simulink subsystem "PvtSubSys_VSM_LCKIE"  (R2020b)
settings: Solver=VariableStepAuto  StartTime=0.0  StopTime=10.0  RelTol=1e-3
values from neighbouring files (symbols this model uses):
  P_VSM_LCKIE_ClassInput = 0.0    [LCKIE.sldd]
  P_VSM_LCKIE_Laneoffset : value not decoded    [LCKIE.sldd]
  P_VSM_LCKIE_Laneoffset_BP : value not decoded    [LCKIE.sldd]
  P_VSM_LCKIE_LatC_DisOffofLanWidth : value not decoded    [LCKIE.sldd]
  P_VSM_LCKIE_LatC_DisOffofSpd : value not decoded    [LCKIE.sldd]
  P_VSM_LCKIE_LatC_DisSW = 0.0    [LCKIE.sldd]
  P_VSM_LCKIE_LatC_LanWidth : value not decoded    [LCKIE.sldd]
  P_VSM_LCKIE_LATC_LimitDis : value not decoded    [LCKIE.sldd]
  P_VSM_LCKIE_LATC_LimitDis_BP : value not decoded    [LCKIE.sldd]
  P_VSM_LCKIE_LatC_LimitDisEgoToObjSelt = 1.5    [LCKIE.sldd]
  P_VSM_LCKIE_LatC_LimitEgoToOppLane = 0.3    [LCKIE.sldd]
  P_VSM_LCKIE_LatC_maxLimitDisREToLane = 2.5    [LCKIE.sldd]
  P_VSM_LCKIE_LatC_minLimitDisREToLane = 1.2    [LCKIE.sldd]
  P_VSM_LCKIE_LatC_MoveEnableDis = 0.0    [LCKIE.sldd]
  P_VSM_LCKIE_LatC_RESafDis = 0.8    [LCKIE.sldd]
  P_VSM_LCKIE_LatC_SafeDisofLanWidth : value not decoded    [LCKIE.sldd]
  P_VSM_LCKIE_LatC_Spd : value not decoded    [LCKIE.sldd]
  P_VSM_LCKIE_LongC_d1 : value not decoded    [LCKIE.sldd]
  P_VSM_LCKIE_LongC_d2 : value not decoded    [LCKIE.sldd]
  P_VSM_LCKIE_LongC_DetaSpd : value not decoded    [LCKIE.sldd]
  P_VSM_LCKIE_LongC_DirecChangeDis = 20.0    [LCKIE.sldd]
  P_VSM_LCKIE_LongC_FleetOff = 80.0    [LCKIE.sldd]
  P_VSM_LCKIE_LongC_maxDis = 80.0    [LCKIE.sldd]
  P_VSM_LCKIE_LongC_minDis = 50.0    [LCKIE.sldd]
  P_VSM_LCKIE_LongC_ShutDownLongDis = -25.0    [LCKIE.sldd]
  P_VSM_LCKIE_LongC_ShutDownTTC = -4.0    [LCKIE.sldd]
  P_VSM_LCKIE_LongC_Spd : value not decoded    [LCKIE.sldd]
  P_VSM_LCKIE_LongC_toff = 10.0    [LCKIE.sldd]
  P_VSM_LCKIE_OFC_ActDis = 10.0    [LCKIE.sldd]
  P_VSM_LCKIE_OFC_DownDis = 10.0    [LCKIE.sldd]
  P_VSM_LCKIE_OFC_DownTTC = 5.0    [LCKIE.sldd]
  P_VSM_LCKIE_OFC_SafDis = 10.0    [LCKIE.sldd]
  P_VSM_LCKIE_OFC_Toff = 3.0    [LCKIE.sldd]
  P_VSM_LCKIE_ORC_LatDis = 1.8    [LCKIE.sldd]
  P_VSM_LCKIE_ORC_LimitDis1 = -30.0    [LCKIE.sldd]
  P_VSM_LCKIE_ORC_LimitDis2 = -10.0    [LCKIE.sldd]
  P_VSM_LCKIE_ORC_LimitTTC = 10.0    [LCKIE.sldd]
  P_VSM_LCKIE_ORC_LowSpd = -5.0    [LCKIE.sldd]
  P_VSM_LCKIE_POC_Delaytime : value not decoded    [LCKIE.sldd]
  P_VSM_LCKIE_POC_detaSpd : value not decoded    [LCKIE.sldd]
  P_VSM_LCKIE_POC_LimitDis = -15.0    [LCKIE.sldd]
  P_VSM_LCKIE_POC_LimitTTC = 2.0    [LCKIE.sldd]
  P_VSM_LCKIE_State_CurveMax = 0.005    [LCKIE.sldd]
  P_VSM_LCKIE_State_CurveMin = 0.0055555555555555558    [LCKIE.sldd]
  P_VSM_LCKIE_State_detaspd = 1.39    [LCKIE.sldd]
  P_VSM_LCKIE_State_detaspd_enable = 1.0    [LCKIE.sldd]
  P_VSM_LCKIE_State_DriverInputTrqValue_enable = 1.0    [LCKIE.sldd]
  P_VSM_LCKIE_State_ELKObjClc = 1.0    [LCKIE.sldd]
  P_VSM_LCKIE_State_HWASts_disable = 1.0    [LCKIE.sldd]
  P_VSM_LCKIE_State_IEObjClc = 1.0    [LCKIE.sldd]
  P_VSM_LCKIE_State_IFVReady = 1.0    [LCKIE.sldd]
  P_VSM_LCKIE_State_lamb_enable = 1.0    [LCKIE.sldd]
  P_VSM_LCKIE_State_Lanecurve_enable = 1.0    [LCKIE.sldd]
  P_VSM_LCKIE_State_LaneWidth_enable = 1.0    [LCKIE.sldd]
  P_VSM_LCKIE_State_Off2on = 3.0    [LCKIE.sldd]
  P_VSM_LCKIE_State_OppObjClc = 1.0    [LCKIE.sldd]
  P_VSM_LCKIE_STATE_ORCObjenable = 0.0    [LCKIE.sldd]
  P_VSM_LCKIE_State_Vehspeed_enable = 1.0    [LCKIE.sldd]
  P_VSM_LCKIE_State_wiper_enable = 1.0    [LCKIE.sldd]
  P_VSM_LCKIE_tcycle = 0.02    [LCKIE.sldd]
undefined symbols (not defined in the file or in its folder): P_Global_Vehicle_Length_m, P_Global_VehicleWidthMin_m, P_VSM_LSMC_SampleTime, STATE
libraries: simulink x62
(part 5 of 5)

== matlab function PvtSubSys_VSM_LCKIE/LCKIE/LCKIE_StateMachine/Subsystem/MATLAB Function ==
  data: DelayReady output uint8; IEAct input boolean; flg output uint8; IEActK1 input boolean; tcycle input single; t_offset input single; flgK1 input uint8; delaytimeK1 input single; delaytime output single
function [DelayReady,flg,delaytime] = fcn(IEAct,IEActK1,tcycle,t_offset,flgK1,delaytimeK1)

flg = uint8(0);
delaytime = single(0);
DelayReady = uint8(1);


if IEAct==0 && IEActK1==1
    flg = uint8(1);
    delaytime = tcycle;
    DelayReady = uint8(0);
end
if flgK1==1
    delaytime = delaytimeK1 + tcycle;
    if delaytime < t_offset
        flg = uint8(1);
        DelayReady = uint8(0);
    end
end

== matlab function PvtSubSys_VSM_LCKIE/LCKIE/Subsystem1/LCKIE_SignalProcess1/IE_LATC/MATLAB Function2 ==
  data: Direct input uint8; latflg input uint8; latmov input single; movdis output single; t_s output single; detaDis output single; Dis2Obj input single; ORCID input uint8; SelctID input uint8; ORCReady input uint8; ORCReadyK1 input uint8; IEAct input boolean; limitDis input single; flgK1 input uint8; flg output uint8; t_disK1 input single; t_dis output single; t_disORK1 input single; t_disOR output single
function [movdis,t_s,detaDis,flg,t_dis,t_disOR] = fcn(Direct,latflg,latmov,Dis2Obj,ORCID,SelctID,ORCReady,ORCReadyK1,IEAct,limitDis,flgK1,t_disK1,t_disORK1)

detaDis = single(0);
movdis = latmov;
flg = uint8(0);
t_s = single(0);
t_dis = single(0);
t_disOR= single(0);
if IEAct==1
    if SelctID > 0
        t_dis = single(Dis2Obj(SelctID));
    else
        t_dis = t_disK1;
    end    
    flg = flgK1;
    if ORCReady==0 && (ORCReadyK1==1 ||flgK1==1)
        flg = uint8(1);
    end
    if ORCReady==1 && ORCReadyK1==0 
        flg = uint8(0);
    end
end

if flg==1
    if ORCID > 0
        t_disOR = single(Dis2Obj(ORCID));
    else
        t_disOR = single(t_disORK1);
    end
    t_s = round((t_disOR+t_dis)*5)/10;
    if latflg == 1
        if abs(t_s)<latmov
            if Direct==1 && t_s<0
                movdis = latmov +t_s;
            elseif Direct==1 && t_s >0
                movdis = latmov - t_s;
            end
        else
            if Direct==1
                if t_s > 0
                    movdis = latmov;
                else
                    detaDis = abs(t_s + latmov);
                    movdis = limitDis;
                end
            else
                if t_s < 0
                    movdis = latmov;
                else
                    detaDis = abs(t_s - latmov);
                    movdis = limitDis;
                end
            end
        end
    end
end

== matlab function PvtSubSys_VSM_LCKIE/LCKIE/Subsystem1/LCKIE_SignalProcess1/IE_OS/OS1 ==
  data: IEACTK1 input boolean; IEState input uint8; ObjNum input uint8; t_Ego2Left input single; t_Ego2Right input single; ObjID input uint8; OppFObjID output uint8; ObjLongPos input single; ObjLatPos input single; ObjWidth input single; ObjFuType input uint8; ObjVx input single; ObjClass input uint8; VheSpd_ms input single; C_valid input boolean; C_A0 input single; C_A1 input single; C_A2 input single; C_A3 input single; L_valid input boolean; L_A0 input single; L_A1 input single; L_A2 input single; L_A3 input single; R_valid input boolean; R_A0 input single; R_A1 input single; R_A2 input single; R_A3 input single; classinput input; ObjIDSelectK1 input uint8; CouterK1 input uint8; Couter1K1 input uint8; OppRObjID output uint8; POSRObjID output uint8; DisEgo2ObjSelect output single; DisEgoToObj output; DetaSpdSelect output single; DisEgo2OppLane output single; DetaSpd output single; ObjLane output uint8; TTC output single; ObjSelectID output uint8; ObjIDSelect output uint8; Couter output uint8; Couter1 output uint8
function [OppFObjID,OppRObjID,POSRObjID,DisEgo2ObjSelect,DisEgoToObj,DetaSpdSelect,DisEgo2OppLane,DetaSpd,ObjLane,TTC,...
    ObjSelectID,ObjIDSelect,Couter,Couter1] = fcn(IEACTK1,IEState,ObjNum,t_Ego2Left,t_Ego2Right,ObjID,...
    ObjLongPos,ObjLatPos,ObjWidth,ObjFuType,ObjVx,ObjClass,VheSpd_ms,C_valid,C_A0,C_A1,C_A2,C_A3,...
    L_valid,L_A0,L_A1,L_A2,L_A3,R_valid,R_A0,R_A1,R_A2,R_A3,classinput,ObjIDSelectK1,CouterK1,Couter1K1)

ObjLane = uint8(zeros(9,1));
DetaSpd = single(zeros(9,1));
TTC = single(255*zeros(9,1));
ObjMovDir = uint8(zeros(9,1));
DisEgoToObj = single(255*zeros(9,1));
OppFObjID = uint8(0);
OppRObjID = uint8(0);
POSRObjID = uint8(0);
DisEgo2ObjSelect = single(0);
DetaSpdSelect =  single(0);
DisEgo2OppLane =  single(0);
ObjSelectID = uint8(0);
ObjIDSelect = uint8(0);
Couter = uint8(0);
Couter1 = uint8(0);

minLFObjDis = single(255);
minRFObjDis = single(255);
minEgoFDis = single(255);
minLFTruckDis = single(255);
minRFTruckDis = single(255);
minLRDis = single(255);
minRRDis = single(255);
minLFObjID = uint8(0);
minRFObjID = uint8(0);
minEgoFID = uint8(0);
minLFTruckID = uint8(0);
minRFTruckID = uint8(0);
minLRID = uint8(0);
minRRID = uint8(0);

for i=1:ObjNum
    %%
    if ObjID(i) == ObjIDSelectK1
        outoff = single(3.5);
        long1 = single(-110);
        long2 = single(130);
        LongSt = single(0);
        DirectSpd = single(-0.65);
    else
        outoff = single(3.3);
        long1 = single(-100);
        long2 = single(120);
        LongSt = single(1);
        DirectSpd = single(-0.25);
    end
    %% 目标属性提取，后方目标针对弯道情况，借用LM相关位置进行分类
    t_x = ObjLongPos(i);
    t_y = ObjLatPos(i);
    t_w = ObjWidth(i)/2;
    if ObjID(i) >0 && t_x >long1 &&  t_x < long2 && ObjFuType(i)~=2
        if t_x >LongSt  %%目标前后位置区分
            ObjLongSts = uint8(1);
        else
            ObjLongSts = uint8(2);
        end
        DetaSpd(i)= -ObjVx(i);
        absObjSpd = single(VheSpd_ms + ObjVx(i)); %%目标运动方向区分
        if absObjSpd > DirectSpd
            ObjMovDir(i) = 1;
        else
            ObjMovDir(i) = 2;
        end
        if abs(ObjVx(i)) > 0.001 %%TTC计算
            TTC(i) = -t_x/ObjVx(i);
        end
        if C_valid >0 && L_valid > 0 && R_valid > 0
            t_Cy = C_A0+C_A1*t_x+C_A2*t_x^2+C_A3*t_x^3;
            if t_y>t_Cy
                t_side = uint8(1); %% Obj in the left of ego vhicle
            else
                t_side = uint8(2);
            end
            if t_side == 1
                t_Ly = L_A0+L_A1*t_x+L_A2*t_x^2+L_A3*t_x^3;
                kL = L_A1+2*L_A2*t_x+3*L_A3*t_x^2;
                t_Lk = sqrt(kL^2+1);
                ObjEdge2Lane = (t_y - t_Ly)/t_Lk - t_w ;
            else
                t_Ry = R_A0+R_A1*t_x+R_A2*t_x^2+R_A3*t_x^3;
                kR = R_A1+2*R_A2*t_x+3*R_A3*t_x^2;
                t_Rk = sqrt(kR^2+1);
                ObjEdge2Lane = (t_Ry - t_y)/t_Rk - t_w ;
            end
            if ObjLongSts == 1
                t_latDis = ObjEdge2Lane + 0.4;
            else
                t_latDis = abs(ObjEdge2Lane);
            end
            if t_latDis <= 0
                ObjLane(i) = uint8(3);
            elseif t_latDis > 0 && t_latDis <= outoff
                if t_side ==1
                    ObjLane(i) = uint8(1);
                    DisEgoToObj(i) = t_Ego2Left + ObjEdge2Lane;
                elseif t_side ==2
                    ObjLane(i) = uint8(2);
                    DisEgoToObj(i) = -(t_Ego2Right + ObjEdge2Lane);
                end
            end
        end
        
        if ObjLongSts == 1
            if ObjLane(i) == 1
                if minLFObjDis >= t_x
                    minLFObjDis = t_x;
                    minLFObjID = uint8(i);
                end
            elseif ObjLane(i) == 2
                if minRFObjDis >= t_x
                    minRFObjDis = t_x;
                    minRFObjID = uint8(i);
                end
            elseif ObjLane(i) == 3
                if minEgoFDis > t_x
                    minEgoFDis = t_x;
                    minEgoFID = uint8(i);
                end
            end
        end
        
        if ObjClass(i) ==3 && ObjLongSts == 1 && ObjMovDir(i) == 1
            if ObjLane(i) == 1
                if minLFTruckDis >= t_x
                    minLFTruckDis = t_x;
                    minLFTruckID = uint8(i);
                end
            elseif ObjLane(i) == 2
                if minRFTruckDis >= t_x
                    minRFTruckDis = t_x;
                    minRFTruckID = uint8(i);
                end
            end
        end
        
        if ObjLongSts == 2 &&ObjMovDir(i) == 1
            if ObjLane(i) == 1
                if minLRDis > abs(t_x)
                    minLRDis = abs(t_x);
                    minLRID = uint8(i);
                end
            elseif ObjLane(i) == 2
                if minRRDis> abs(t_x)
                    minRRDis = abs(t_x);
                    minRRID = uint8(i);
                end
            end
        end
    end
end
%% 主目标筛选，并针对相对速度进行相应延时选择处理
if classinput == 1
    if ObjMovDir(minLFObjID)==1
        minLFTruckID = minLFObjID;
    end
    if  ObjMovDir(minRFObjID)==1
        minRFTruckID = minRFObjID;
    end
end

if minLFTruckID>0 && minRFTruckID >0
    t_h = minLFTruckDis - minRFTruckDis;
    if t_h >0
        t_selectID = minRFTruckID;
    else
        t_selectID = minLFTruckID;
    end
elseif minLFTruckID == 0 && minRFTruckID >0
    t_selectID = minRFTruckID;
elseif minLFTruckID > 0 && minRFTruckID == 0
    t_selectID = minLFTruckID;
else
    t_selectID = uint8(0);
end
if t_selectID >0
    if ObjID(t_selectID) == ObjIDSelectK1
        if DetaSpd(t_selectID) > -1.3
            ObjSelectID = t_selectID;
        else
            Couter = min(CouterK1+uint8(1),uint8(6));
            if Couter <5
                ObjSelectID = t_selectID;
            end
        end
    else
        if  DetaSpd(t_selectID) >0.1
            Couter1 = min(Couter1K1+uint8(1),uint8(16));
            if Couter1 >10
                ObjSelectID = t_selectID;
            end
        end
    end
end
%%
if ObjSelectID >0
    if ObjLane(ObjSelectID) == 1
        DisEgo2OppLane = t_Ego2Right;
        OppFObjID = minRFObjID;
        OppRObjID = minRRID;
        POSRObjID = minLRID;
    elseif ObjLane(ObjSelectID) == 2
        DisEgo2OppLane = t_Ego2Left;
        OppFObjID = minLFObjID;
        OppRObjID = minLRID;
        POSRObjID = minRRID;
    end
else
    if IEACTK1==1
        if IEState == 5
            DisEgo2OppLane = t_Ego2Left;
            OppFObjID = minLFObjID;
            OppRObjID = minLRID;
            POSRObjID = minRRID;
        elseif IEState == 4
            DisEgo2OppLane = t_Ego2Right;
            OppFObjID = minRFObjID;
            OppRObjID = minRRID;
            POSRObjID = minLRID;
        end
    end
end
if ObjSelectID >0
    DisEgo2ObjSelect = abs(DisEgoToObj(ObjSelectID));
    DetaSpdSelect =  DetaSpd(ObjSelectID);
    ObjIDSelect = ObjID(ObjSelectID);
end

== stateflow chart PvtSubSys_VSM_LCKIE/LCKIE/LCKIE_StateMachine/LCKIE_State ==
  state MAINST_OFF
    en:State=STATE.OFF;
  state MAINST_ON
    en:State=STATE.ERROR;
  state enabled
    state IDLE
      en:State=STATE.IDLE
    state MAINST_ON
      en:State=STATE.READY;
    state ACTIVE
      state right
        en:State=STATE.ACTIVE_LEFT;
      state left
        en:State=STATE.ACTIVE_RIGHT;
      state active
        en:State=STATE.ACTIVE;
      active -> left [order 2] : [LCKIEleft==1&&HWAready ==1]
      active -> right [order 1] : [LCKIEright==1&&HWAready ==1]
      left -> active : [HWAready ==0]
      right -> active : [HWAready == 0]
    (default) -> IDLE
    IDLE -> enabled.MAINST_ON : [LCKSTATE==true&&...
        | IE_Idel2Ready]
    enabled.MAINST_ON -> IDLE [order 1] : [IE_Ready2Idel||...
        | LCKSTATE==false]
    ACTIVE -> IDLE [order 2] : [IE_Ready2Idel||...
        | LCKSTATE==false]
    enabled.MAINST_ON -> active [order 2] : [IE_Ready2Active&&...
        | DelayReady==1]
    ACTIVE -> enabled.MAINST_ON [order 1] : [IE_Active2Ready]
  (default) -> MAINST_OFF
  MAINST_OFF -> MAINST_ON [order 2] : [IntelligentEvaSwtReq==true  &&...
      |  VehConfigLCKIE==1&&IFV_Fail]
  MAINST_ON -> MAINST_OFF : [IntelligentEvaSwtReq==false]
  MAINST_OFF -> enabled [order 1] : [IntelligentEvaSwtReq==true  &&...
      |  VehConfigLCKIE==1&&...
      | IFV_Enable]
  enabled -> MAINST_OFF [order 1] : [IntelligentEvaSwtReq==false]
  enabled -> MAINST_ON [order 2] : [IFV_Fail]
  data: IntelligentEvaSwtReq input boolean; VehConfigLCKIE input uint8; LCKSTATE input boolean; IE_Idel2Ready input boolean; IE_Ready2Active input boolean; IE_Ready2Idel input boolean; IE_Active2Ready input boolean; HWAready input boolean; IFV_Enable input boolean; IFV_Fail input boolean; DelayReady input uint8; LCKIEleft input boolean; LCKIEright input boolean; State output Enum: STATE =STATE.OFF
